simulink model "fft_overlap_tomori"  (R2023b)
settings: Solver=VariableStepAuto  StartTime=0.0  StopTime=inf  RelTol=1e-3
InitFcn:
  | fftparrallelout
  | load('dataram.mat')
  | s= fi(exp(-1j*2*pi.*(0:63)/64),1,16,15);
  | fixed_point = fixdt(1,27,20);
  | fixed_pointu = fixdt(0,29,20);
  | fixed = fixdt(1,22,15);
  | const = fixdt(1,18,17);
  | addConst = fixdt(1,18,16);
  | f =10.4e6;
  | f1=45e6;
  | alpha1 =5;
  | beta1 = 0.00001 ;
  | beta2 = 0.99999 ;
  | beta3 = 23;
undefined symbols (not defined in the file or in its folder): j
libraries: dspxfrm3 x11, commrflib2 x4
(part 8 of 10)

== system fft_overlap_tomori/FFT64_outMuxed/64pointFFTchan/FFT64/FFT32_1/complexmult4 ==
  x1 : Inport
  In3 : Inport  Port=2
  Add1 : Sum  OutDataTypeStr=addConst  RndMeth=Round
  Add2 : Sum  Inputs=+-  OutDataTypeStr=fixed  AccumDataTypeStr=fixed  RndMeth=Round
  Add20 : Sum  OutDataTypeStr=fixed  RndMeth=Round
  Add3 : Sum  Inputs=+-  OutDataTypeStr=fixed  AccumDataTypeStr=fixed  RndMeth=Round
  Add4 : Sum  Inputs=+-  OutDataTypeStr=fixed  AccumDataTypeStr=fixed  RndMeth=Round
  Complex to Real-Imag : ComplexToRealImag
  Complex to Real-Imag1 : ComplexToRealImag
  Constant : Constant  Commented=on  Value=1+j  OutDataTypeStr=fixdt(1,22, 15)  SampleTime=2e-8
  Constant1 : Constant  Commented=on  Value=1-j  OutDataTypeStr=fixdt(1,22, 15)  SampleTime=2e-8
  Data Type Conversion : DataTypeConversion  OutDataTypeStr=fixed  RndMeth=Round  SaturateOnIntegerOverflow=off
  Data Type Conversion1 : DataTypeConversion  OutDataTypeStr=fixed  RndMeth=Round  SaturateOnIntegerOverflow=off
  Data Type Conversion2 : DataTypeConversion  OutDataTypeStr=fixed  RndMeth=Round  SaturateOnIntegerOverflow=off
  Delay : Delay
  Delay1 : Delay
  Delay{3..14} (12 alike) : Delay  DelayLength=1
  Delay2 : Delay
  Display : Display  Commented=on
  Product : Product
  Product1 : Product
  Product2 : Product
  Real-Imag to Complex : RealImagToComplex
  Out1 : Outport
  wires:
  Real-Imag to Complex/1 -> Out1/1
  In3/1 -> Complex to Real-Imag1/1
  x1/1 -> Complex to Real-Imag/1
  Product/1 -> Delay/1
  Product1/1 -> Delay1/1
  Product2/1 -> Delay2/1
  Delay/1 -> Data Type Conversion/1
  Delay1/1 -> Data Type Conversion1/1
  Delay2/1 -> Data Type Conversion2/1
  Add4/1 -> Delay9/1
  Add3/1 -> Delay10/1
  Add20/1 -> Delay3/1
  Add1/1 -> Delay4/1
  Complex to Real-Imag/1 -> Delay5/1, Add20/1
  Complex to Real-Imag1/1 -> Delay6/1, Add1/1
  Complex to Real-Imag/2 -> Delay7/1, Add20/2
  Complex to Real-Imag1/2 -> Delay8/1, Add1/2
  Delay3/1 -> Product/1
  Delay4/1 -> Product/2
  Delay5/1 -> Product1/1
  Delay6/1 -> Product1/2
  Delay7/1 -> Product2/1
  Delay8/1 -> Product2/2
  Delay9/1 -> Real-Imag to Complex/1
  Delay10/1 -> Add2/1
  Delay11/1 -> Add2/2
  Add2/1 -> Real-Imag to Complex/2
  Delay12/1 -> Add3/1
  Data Type Conversion/1 -> Delay12/1
  Data Type Conversion1/1 -> Delay13/1
  Delay13/1 -> Add4/1, Add3/2
  Data Type Conversion2/1 -> Delay14/1
  Delay14/1 -> Delay11/1, Add4/2

== system fft_overlap_tomori/FFT64_outMuxed/64pointFFTchan/FFT64/FFT32_1/complexmult5 ==
  x1 : Inport
  In3 : Inport  Port=2
  Add1 : Sum  OutDataTypeStr=addConst  RndMeth=Round
  Add2 : Sum  Inputs=+-  OutDataTypeStr=fixed  AccumDataTypeStr=fixed  RndMeth=Round
  Add20 : Sum  OutDataTypeStr=fixed  RndMeth=Round
  Add3 : Sum  Inputs=+-  OutDataTypeStr=fixed  AccumDataTypeStr=fixed  RndMeth=Round
  Add4 : Sum  Inputs=+-  OutDataTypeStr=fixed  AccumDataTypeStr=fixed  RndMeth=Round
  Complex to Real-Imag : ComplexToRealImag
  Complex to Real-Imag1 : ComplexToRealImag
  Constant : Constant  Commented=on  Value=1+j  OutDataTypeStr=fixdt(1,22, 15)  SampleTime=2e-8
  Constant1 : Constant  Commented=on  Value=1-j  OutDataTypeStr=fixdt(1,22, 15)  SampleTime=2e-8
  Data Type Conversion : DataTypeConversion  OutDataTypeStr=fixed  RndMeth=Round  SaturateOnIntegerOverflow=off
  Data Type Conversion1 : DataTypeConversion  OutDataTypeStr=fixed  RndMeth=Round  SaturateOnIntegerOverflow=off
  Data Type Conversion2 : DataTypeConversion  OutDataTypeStr=fixed  RndMeth=Round  SaturateOnIntegerOverflow=off
  Delay : Delay
  Delay1 : Delay
  Delay{3..14} (12 alike) : Delay  DelayLength=1
  Delay2 : Delay
  Display : Display  Commented=on
  Product : Product
  Product1 : Product
  Product2 : Product
  Real-Imag to Complex : RealImagToComplex
  Out1 : Outport
  wires:
  Delay14/1 -> Add4/2, Delay11/1
  Data Type Conversion2/1 -> Delay14/1
  Delay13/1 -> Add3/2, Add4/1
  Data Type Conversion1/1 -> Delay13/1
  Data Type Conversion/1 -> Delay12/1
  Delay12/1 -> Add3/1
  Add2/1 -> Real-Imag to Complex/2
  Delay11/1 -> Add2/2
  Delay10/1 -> Add2/1
  Delay9/1 -> Real-Imag to Complex/1
  Delay8/1 -> Product2/2
  Delay7/1 -> Product2/1
  Delay6/1 -> Product1/2
  Delay5/1 -> Product1/1
  Delay4/1 -> Product/2
  Delay3/1 -> Product/1
  Complex to Real-Imag1/2 -> Add1/2, Delay8/1
  Complex to Real-Imag/2 -> Add20/2, Delay7/1
  Complex to Real-Imag1/1 -> Add1/1, Delay6/1
  Complex to Real-Imag/1 -> Add20/1, Delay5/1
  Add1/1 -> Delay4/1
  Add20/1 -> Delay3/1
  Add3/1 -> Delay10/1
  Add4/1 -> Delay9/1
  Delay2/1 -> Data Type Conversion2/1
  Delay1/1 -> Data Type Conversion1/1
  Delay/1 -> Data Type Conversion/1
  Product2/1 -> Delay2/1
  Product1/1 -> Delay1/1
  Product/1 -> Delay/1
  x1/1 -> Complex to Real-Imag/1
  In3/1 -> Complex to Real-Imag1/1
  Real-Imag to Complex/1 -> Out1/1

== system fft_overlap_tomori/FFT64_outMuxed/64pointFFTchan/FFT64/FFT32_1/complexmult6 ==
  x1 : Inport
  In3 : Inport  Port=2
  Add1 : Sum  OutDataTypeStr=addConst  RndMeth=Round
  Add2 : Sum  Inputs=+-  OutDataTypeStr=fixed  AccumDataTypeStr=fixed  RndMeth=Round
  Add20 : Sum  OutDataTypeStr=fixed  RndMeth=Round
  Add3 : Sum  Inputs=+-  OutDataTypeStr=fixed  AccumDataTypeStr=fixed  RndMeth=Round
  Add4 : Sum  Inputs=+-  OutDataTypeStr=fixed  AccumDataTypeStr=fixed  RndMeth=Round
  Complex to Real-Imag : ComplexToRealImag
  Complex to Real-Imag1 : ComplexToRealImag
  Constant : Constant  Commented=on  Value=1+j  OutDataTypeStr=fixdt(1,22, 15)  SampleTime=2e-8
  Constant1 : Constant  Commented=on  Value=1-j  OutDataTypeStr=fixdt(1,22, 15)  SampleTime=2e-8
  Data Type Conversion : DataTypeConversion  OutDataTypeStr=fixed  RndMeth=Round  SaturateOnIntegerOverflow=off
  Data Type Conversion1 : DataTypeConversion  OutDataTypeStr=fixed  RndMeth=Round  SaturateOnIntegerOverflow=off
  Data Type Conversion2 : DataTypeConversion  OutDataTypeStr=fixed  RndMeth=Round  SaturateOnIntegerOverflow=off
  Delay : Delay
  Delay1 : Delay
  Delay{3..14} (12 alike) : Delay  DelayLength=1
  Delay2 : Delay
  Display : Display  Commented=on
  Product : Product
  Product1 : Product
  Product2 : Product
  Real-Imag to Complex : RealImagToComplex
  Out1 : Outport
  wires:
  Real-Imag to Complex/1 -> Out1/1
  In3/1 -> Complex to Real-Imag1/1
  x1/1 -> Complex to Real-Imag/1
  Product/1 -> Delay/1
  Product1/1 -> Delay1/1
  Product2/1 -> Delay2/1
  Delay/1 -> Data Type Conversion/1
  Delay1/1 -> Data Type Conversion1/1
  Delay2/1 -> Data Type Conversion2/1
  Add4/1 -> Delay9/1
  Add3/1 -> Delay10/1
  Add20/1 -> Delay3/1
  Add1/1 -> Delay4/1
  Complex to Real-Imag/1 -> Delay5/1, Add20/1
  Complex to Real-Imag1/1 -> Delay6/1, Add1/1
  Complex to Real-Imag/2 -> Delay7/1, Add20/2
  Complex to Real-Imag1/2 -> Delay8/1, Add1/2
  Delay3/1 -> Product/1
  Delay4/1 -> Product/2
  Delay5/1 -> Product1/1
  Delay6/1 -> Product1/2
  Delay7/1 -> Product2/1
  Delay8/1 -> Product2/2
  Delay9/1 -> Real-Imag to Complex/1
  Delay10/1 -> Add2/1
  Delay11/1 -> Add2/2
  Add2/1 -> Real-Imag to Complex/2
  Delay12/1 -> Add3/1
  Data Type Conversion/1 -> Delay12/1
  Data Type Conversion1/1 -> Delay13/1
  Delay13/1 -> Add4/1, Add3/2
  Data Type Conversion2/1 -> Delay14/1
  Delay14/1 -> Delay11/1, Add4/2

== system fft_overlap_tomori/FFT64_outMuxed/64pointFFTchan/FFT64/FFT32_1/complexmult7 ==
  x1 : Inport
  In3 : Inport  Port=2
  Add1 : Sum  OutDataTypeStr=addConst  RndMeth=Round
  Add2 : Sum  Inputs=+-  OutDataTypeStr=fixed  AccumDataTypeStr=fixed  RndMeth=Round
  Add20 : Sum  OutDataTypeStr=fixed  RndMeth=Round
  Add3 : Sum  Inputs=+-  OutDataTypeStr=fixed  AccumDataTypeStr=fixed  RndMeth=Round
  Add4 : Sum  Inputs=+-  OutDataTypeStr=fixed  AccumDataTypeStr=fixed  RndMeth=Round
  Complex to Real-Imag : ComplexToRealImag
  Complex to Real-Imag1 : ComplexToRealImag
  Constant : Constant  Commented=on  Value=1+j  OutDataTypeStr=fixdt(1,22, 15)  SampleTime=2e-8
  Constant1 : Constant  Commented=on  Value=1-j  OutDataTypeStr=fixdt(1,22, 15)  SampleTime=2e-8
  Data Type Conversion : DataTypeConversion  OutDataTypeStr=fixed  RndMeth=Round  SaturateOnIntegerOverflow=off
  Data Type Conversion1 : DataTypeConversion  OutDataTypeStr=fixed  RndMeth=Round  SaturateOnIntegerOverflow=off
  Data Type Conversion2 : DataTypeConversion  OutDataTypeStr=fixed  RndMeth=Round  SaturateOnIntegerOverflow=off
  Delay : Delay
  Delay1 : Delay
  Delay{3..14} (12 alike) : Delay  DelayLength=1
  Delay2 : Delay
  Display : Display  Commented=on
  Product : Product
  Product1 : Product
  Product2 : Product
  Real-Imag to Complex : RealImagToComplex
  Out1 : Outport
  wires:
  Delay14/1 -> Add4/2, Delay11/1
  Data Type Conversion2/1 -> Delay14/1
  Delay13/1 -> Add3/2, Add4/1
  Data Type Conversion1/1 -> Delay13/1
  Data Type Conversion/1 -> Delay12/1
  Delay12/1 -> Add3/1
  Add2/1 -> Real-Imag to Complex/2
  Delay11/1 -> Add2/2
  Delay10/1 -> Add2/1
  Delay9/1 -> Real-Imag to Complex/1
  Delay8/1 -> Product2/2
  Delay7/1 -> Product2/1
  Delay6/1 -> Product1/2
  Delay5/1 -> Product1/1
  Delay4/1 -> Product/2
  Delay3/1 -> Product/1
  Complex to Real-Imag1/2 -> Add1/2, Delay8/1
  Complex to Real-Imag/2 -> Add20/2, Delay7/1
  Complex to Real-Imag1/1 -> Add1/1, Delay6/1
  Complex to Real-Imag/1 -> Add20/1, Delay5/1
  Add1/1 -> Delay4/1
  Add20/1 -> Delay3/1
  Add3/1 -> Delay10/1
  Add4/1 -> Delay9/1
  Delay2/1 -> Data Type Conversion2/1
  Delay1/1 -> Data Type Conversion1/1
  Delay/1 -> Data Type Conversion/1
  Product2/1 -> Delay2/1
  Product1/1 -> Delay1/1
  Product/1 -> Delay/1
  x1/1 -> Complex to Real-Imag/1
  In3/1 -> Complex to Real-Imag1/1
  Real-Imag to Complex/1 -> Out1/1

== system fft_overlap_tomori/FFT64_outMuxed/64pointFFTchan/FFT64/FFT32_1/complexmult8 ==
  x1 : Inport
  In3 : Inport  Port=2
  Add1 : Sum  OutDataTypeStr=addConst  RndMeth=Round
  Add2 : Sum  Inputs=+-  OutDataTypeStr=fixed  AccumDataTypeStr=fixed  RndMeth=Round
  Add20 : Sum  OutDataTypeStr=fixed  RndMeth=Round
  Add3 : Sum  Inputs=+-  OutDataTypeStr=fixed  AccumDataTypeStr=fixed  RndMeth=Round
  Add4 : Sum  Inputs=+-  OutDataTypeStr=fixed  AccumDataTypeStr=fixed  RndMeth=Round
  Complex to Real-Imag : ComplexToRealImag
  Complex to Real-Imag1 : ComplexToRealImag
  Constant : Constant  Commented=on  Value=1+j  OutDataTypeStr=fixdt(1,22, 15)  SampleTime=2e-8
  Constant1 : Constant  Commented=on  Value=1-j  OutDataTypeStr=fixdt(1,22, 15)  SampleTime=2e-8
  Data Type Conversion : DataTypeConversion  OutDataTypeStr=fixed  RndMeth=Round  SaturateOnIntegerOverflow=off
  Data Type Conversion1 : DataTypeConversion  OutDataTypeStr=fixed  RndMeth=Round  SaturateOnIntegerOverflow=off
  Data Type Conversion2 : DataTypeConversion  OutDataTypeStr=fixed  RndMeth=Round  SaturateOnIntegerOverflow=off
  Delay : Delay
  Delay1 : Delay
  Delay{3..14} (12 alike) : Delay  DelayLength=1
  Delay2 : Delay
  Display : Display  Commented=on
  Product : Product
  Product1 : Product
  Product2 : Product
  Real-Imag to Complex : RealImagToComplex
  Out1 : Outport
  wires:
  Real-Imag to Complex/1 -> Out1/1
  In3/1 -> Complex to Real-Imag1/1
  x1/1 -> Complex to Real-Imag/1
  Product/1 -> Delay/1
  Product1/1 -> Delay1/1
  Product2/1 -> Delay2/1
  Delay/1 -> Data Type Conversion/1
  Delay1/1 -> Data Type Conversion1/1
  Delay2/1 -> Data Type Conversion2/1
  Add4/1 -> Delay9/1
  Add3/1 -> Delay10/1
  Add20/1 -> Delay3/1
  Add1/1 -> Delay4/1
  Complex to Real-Imag/1 -> Delay5/1, Add20/1
  Complex to Real-Imag1/1 -> Delay6/1, Add1/1
  Complex to Real-Imag/2 -> Delay7/1, Add20/2
  Complex to Real-Imag1/2 -> Delay8/1, Add1/2
  Delay3/1 -> Product/1
  Delay4/1 -> Product/2
  Delay5/1 -> Product1/1
  Delay6/1 -> Product1/2
  Delay7/1 -> Product2/1
  Delay8/1 -> Product2/2
  Delay9/1 -> Real-Imag to Complex/1
  Delay10/1 -> Add2/1
  Delay11/1 -> Add2/2
  Add2/1 -> Real-Imag to Complex/2
  Delay12/1 -> Add3/1
  Data Type Conversion/1 -> Delay12/1
  Data Type Conversion1/1 -> Delay13/1
  Delay13/1 -> Add4/1, Add3/2
  Data Type Conversion2/1 -> Delay14/1
  Delay14/1 -> Delay11/1, Add4/2

== system fft_overlap_tomori/FFT64_outMuxed/64pointFFTchan/FFT64/FFT32_1/complexmult9 ==
  x1 : Inport
  In3 : Inport  Port=2
  Add1 : Sum  OutDataTypeStr=addConst  RndMeth=Round
  Add2 : Sum  Inputs=+-  OutDataTypeStr=fixed  AccumDataTypeStr=fixed  RndMeth=Round
  Add20 : Sum  OutDataTypeStr=fixed  RndMeth=Round
  Add3 : Sum  Inputs=+-  OutDataTypeStr=fixed  AccumDataTypeStr=fixed  RndMeth=Round
  Add4 : Sum  Inputs=+-  OutDataTypeStr=fixed  AccumDataTypeStr=fixed  RndMeth=Round
  Complex to Real-Imag : ComplexToRealImag
  Complex to Real-Imag1 : ComplexToRealImag
  Constant : Constant  Commented=on  Value=1+j  OutDataTypeStr=fixdt(1,22, 15)  SampleTime=2e-8
  Constant1 : Constant  Commented=on  Value=1-j  OutDataTypeStr=fixdt(1,22, 15)  SampleTime=2e-8
  Data Type Conversion : DataTypeConversion  OutDataTypeStr=fixed  RndMeth=Round  SaturateOnIntegerOverflow=off
  Data Type Conversion1 : DataTypeConversion  OutDataTypeStr=fixed  RndMeth=Round  SaturateOnIntegerOverflow=off
  Data Type Conversion2 : DataTypeConversion  OutDataTypeStr=fixed  RndMeth=Round  SaturateOnIntegerOverflow=off
  Delay : Delay
  Delay1 : Delay
  Delay{3..14} (12 alike) : Delay  DelayLength=1
  Delay2 : Delay
  Display : Display  Commented=on
  Product : Product
  Product1 : Product
  Product2 : Product
  Real-Imag to Complex : RealImagToComplex
  Out1 : Outport
  wires:
  Delay14/1 -> Add4/2, Delay11/1
  Data Type Conversion2/1 -> Delay14/1
  Delay13/1 -> Add3/2, Add4/1
  Data Type Conversion1/1 -> Delay13/1
  Data Type Conversion/1 -> Delay12/1
  Delay12/1 -> Add3/1
  Add2/1 -> Real-Imag to Complex/2
  Delay11/1 -> Add2/2
  Delay10/1 -> Add2/1
  Delay9/1 -> Real-Imag to Complex/1
  Delay8/1 -> Product2/2
  Delay7/1 -> Product2/1
  Delay6/1 -> Product1/2
  Delay5/1 -> Product1/1
  Delay4/1 -> Product/2
  Delay3/1 -> Product/1
  Complex to Real-Imag1/2 -> Add1/2, Delay8/1
  Complex to Real-Imag/2 -> Add20/2, Delay7/1
  Complex to Real-Imag1/1 -> Add1/1, Delay6/1
  Complex to Real-Imag/1 -> Add20/1, Delay5/1
  Add1/1 -> Delay4/1
  Add20/1 -> Delay3/1
  Add3/1 -> Delay10/1
  Add4/1 -> Delay9/1
  Delay2/1 -> Data Type Conversion2/1
  Delay1/1 -> Data Type Conversion1/1
  Delay/1 -> Data Type Conversion/1
  Product2/1 -> Delay2/1
  Product1/1 -> Delay1/1
  Product/1 -> Delay/1
  x1/1 -> Complex to Real-Imag/1
  In3/1 -> Complex to Real-Imag1/1
  Real-Imag to Complex/1 -> Out1/1

== system fft_overlap_tomori/FFT64_outMuxed/64pointFFTchan/FFT64/FFT32_1/multByExp(-j*Pi//4) ==
  x4 : Inport
  Add : Sum  OutDataTypeStr=fixed  RndMeth=Round
  Add1 : Sum  Inputs=+-  OutDataTypeStr=fixed  RndMeth=Round
  Complex to Real-Imag : ComplexToRealImag
  Data Type Conversion : DataTypeConversion  OutDataTypeStr=fixed  RndMeth=Round  SaturateOnIntegerOverflow=off
  Delay1 : Delay  DelayLength=1
  Delay24 : Delay  DelayLength=1
  Gain : Gain  Gain=sqrt(2)/2  ParamDataTypeStr=const
  Real-Imag to Complex : RealImagToComplex
  Out1 : Outport
  wires:
  x4/1 -> Gain/1
  Real-Imag to Complex/1 -> Out1/1
  Delay24/1 -> Complex to Real-Imag/1
  Add1/1 -> Real-Imag to Complex/2
  Add/1 -> Real-Imag to Complex/1
  Complex to Real-Imag/2 -> Add/2, Add1/1
  Complex to Real-Imag/1 -> Add/1, Add1/2
  Gain/1 -> Delay1/1
  Delay1/1 -> Data Type Conversion/1
  Data Type Conversion/1 -> Delay24/1

== system fft_overlap_tomori/FFT64_outMuxed/64pointFFTchan/FFT64/FFT32_1/multByExp(-j*Pi//4)1 ==
  x4 : Inport
  Add : Sum  OutDataTypeStr=fixed  RndMeth=Round
  Add1 : Sum  Inputs=+-  OutDataTypeStr=fixed  RndMeth=Round
  Complex to Real-Imag : ComplexToRealImag
  Data Type Conversion : DataTypeConversion  OutDataTypeStr=fixed  RndMeth=Round  SaturateOnIntegerOverflow=off
  Delay1 : Delay  DelayLength=1
  Delay24 : Delay  DelayLength=1
  Gain : Gain  Gain=sqrt(2)/2  ParamDataTypeStr=const
  Real-Imag to Complex : RealImagToComplex
  Out1 : Outport
  wires:
  x4/1 -> Gain/1
  Real-Imag to Complex/1 -> Out1/1
  Delay24/1 -> Complex to Real-Imag/1
  Add1/1 -> Real-Imag to Complex/2
  Add/1 -> Real-Imag to Complex/1
  Complex to Real-Imag/2 -> Add/2, Add1/1
  Complex to Real-Imag/1 -> Add/1, Add1/2
  Gain/1 -> Delay1/1
  Delay1/1 -> Data Type Conversion/1
  Data Type Conversion/1 -> Delay24/1

== system fft_overlap_tomori/FFT64_outMuxed/64pointFFTchan/FFT64/FFT32_1/multByMinusJ ==
  x4 : Inport
  Complex to Real-Imag : ComplexToRealImag
  Real-Imag to Complex : RealImagToComplex
  Unary Minus1 : UnaryMinus
  Out1 : Outport
  wires:
  Complex to Real-Imag/1 -> Unary Minus1/1
  Complex to Real-Imag/2 -> Real-Imag to Complex/1
  x4/1 -> Complex to Real-Imag/1
  Real-Imag to Complex/1 -> Out1/1
  Unary Minus1/1 -> Real-Imag to Complex/2

== system fft_overlap_tomori/FFT64_outMuxed/64pointFFTchan/FFT64/FFT32_1/multByMinusJ3 ==
  In1 : Inport
  Complex to Real-Imag : ComplexToRealImag
  Real-Imag to Complex : RealImagToComplex
  Unary Minus1 : UnaryMinus
  Out1 : Outport
  wires:
  Complex to Real-Imag/1 -> Unary Minus1/1
  Complex to Real-Imag/2 -> Real-Imag to Complex/1
  In1/1 -> Complex to Real-Imag/1
  Real-Imag to Complex/1 -> Out1/1
  Unary Minus1/1 -> Real-Imag to Complex/2

== system fft_overlap_tomori/16//32 and test junk/16pointfftchan1/fft_res/fft_1/proddd/s3 ==
  In1 : Inport
  Add16 : Sum  OutDataTypeStr=fixed_point  AccumDataTypeStr=fixed_point
  Add21 : Sum  Inputs=+-  OutDataTypeStr=fixed_point  AccumDataTypeStr=fixed_point
  Complex to Real-Imag : ComplexToRealImag
  Real-Imag to Complex : RealImagToComplex
  Out1 : Outport  VectorParamsAs1DForOutWhenUnconnected=off
  wires:
  Real-Imag to Complex/1 -> Out1/1
  In1/1 -> Complex to Real-Imag/1
  Complex to Real-Imag/1 -> Add21/2, Add16/1
  Complex to Real-Imag/2 -> Add21/1, Add16/2
  Add16/1 -> Real-Imag to Complex/1
  Add21/1 -> Real-Imag to Complex/2

== system fft_overlap_tomori/16//32 and test junk/16pointfftchan1/fft_res/fft_1/ptrrt/s4 ==
  In1 : Inport
  Add16 : Sum  OutDataTypeStr=fixed_point  AccumDataTypeStr=fixed_point
  Add21 : Sum  Inputs=+-  OutDataTypeStr=fixed_point  AccumDataTypeStr=fixed_point
  Complex to Real-Imag : ComplexToRealImag
  Real-Imag to Complex : RealImagToComplex
  Out1 : Outport  VectorParamsAs1DForOutWhenUnconnected=off
  wires:
  In1/1 -> Complex to Real-Imag/1
  Real-Imag to Complex/1 -> Out1/1
  Complex to Real-Imag/1 -> Add16/1, Add21/1
  Complex to Real-Imag/2 -> Add16/2, Add21/2
  Add21/1 -> Real-Imag to Complex/1
  Add16/1 -> Real-Imag to Complex/2

== system fft_overlap_tomori/16//32 and test junk/16pointfftchan1/fft_res/fft_8/proddd/s3 ==
  In1 : Inport
  Add16 : Sum  OutDataTypeStr=fixed_point  AccumDataTypeStr=fixed_point
  Add21 : Sum  Inputs=+-  OutDataTypeStr=fixed_point  AccumDataTypeStr=fixed_point
  Complex to Real-Imag : ComplexToRealImag
  Real-Imag to Complex : RealImagToComplex
  Out1 : Outport  VectorParamsAs1DForOutWhenUnconnected=off
  wires:
  Add21/1 -> Real-Imag to Complex/2
  Add16/1 -> Real-Imag to Complex/1
  Complex to Real-Imag/2 -> Add16/2, Add21/1
  Complex to Real-Imag/1 -> Add16/1, Add21/2
  In1/1 -> Complex to Real-Imag/1
  Real-Imag to Complex/1 -> Out1/1

== system fft_overlap_tomori/16//32 and test junk/16pointfftchan1/fft_res/fft_8/ptrrt/s4 ==
  In1 : Inport
  Add16 : Sum  OutDataTypeStr=fixed_point  AccumDataTypeStr=fixed_point
  Add21 : Sum  Inputs=+-  OutDataTypeStr=fixed_point  AccumDataTypeStr=fixed_point
  Complex to Real-Imag : ComplexToRealImag
  Real-Imag to Complex : RealImagToComplex
  Out1 : Outport  VectorParamsAs1DForOutWhenUnconnected=off
  wires:
  Add16/1 -> Real-Imag to Complex/2
  Add21/1 -> Real-Imag to Complex/1
  Complex to Real-Imag/2 -> Add21/2, Add16/2
  Complex to Real-Imag/1 -> Add21/1, Add16/1
  Real-Imag to Complex/1 -> Out1/1
  In1/1 -> Complex to Real-Imag/1

== system fft_overlap_tomori/16//32 and test junk/32/FFT32/FFT16/FFT8/multByExp(-j*Pi//4) ==
  In1 : Inport
  Add : Sum  OutDataTypeStr=fixed  RndMeth=Round
  Add1 : Sum  Inputs=+-  OutDataTypeStr=fixed  RndMeth=Round
  Complex to Real-Imag : ComplexToRealImag
  Delay24 : Delay
  Gain : Gain  Gain=sqrt(2)/2  ParamDataTypeStr=fixed  OutDataTypeStr=fixed  RndMeth=Round
  Real-Imag to Complex : RealImagToComplex
  Out1 : Outport
  wires:
  Real-Imag to Complex/1 -> Out1/1
  Gain/1 -> Delay24/1
  Complex to Real-Imag/1 -> Add1/2, Add/1
  Complex to Real-Imag/2 -> Add1/1, Add/2
  Add/1 -> Real-Imag to Complex/1
  Add1/1 -> Real-Imag to Complex/2
  Delay24/1 -> Complex to Real-Imag/1
  In1/1 -> Gain/1

== system fft_overlap_tomori/16//32 and test junk/32/FFT32/FFT16/FFT8/multByExp(-j*Pi//4)1 ==
  In1 : Inport
  Add : Sum  OutDataTypeStr=fixed  RndMeth=Round
  Add1 : Sum  Inputs=+-  OutDataTypeStr=fixed  RndMeth=Round
  Complex to Real-Imag : ComplexToRealImag
  Delay24 : Delay
  Gain : Gain  Gain=sqrt(2)/2  ParamDataTypeStr=fixed  OutDataTypeStr=fixed  RndMeth=Round
  Real-Imag to Complex : RealImagToComplex
  Out1 : Outport
  wires:
  Real-Imag to Complex/1 -> Out1/1
  Gain/1 -> Delay24/1
  Complex to Real-Imag/1 -> Add1/2, Add/1
  Complex to Real-Imag/2 -> Add1/1, Add/2
  Add/1 -> Real-Imag to Complex/1
  Add1/1 -> Real-Imag to Complex/2
  Delay24/1 -> Complex to Real-Imag/1
  In1/1 -> Gain/1

== system fft_overlap_tomori/16//32 and test junk/32/FFT32/FFT16/FFT8/multByMinusJ ==
  In1 : Inport
  Complex to Real-Imag : ComplexToRealImag
  Real-Imag to Complex : RealImagToComplex
  Unary Minus1 : UnaryMinus
  Out1 : Outport
  wires:
  Complex to Real-Imag/1 -> Unary Minus1/1
  Complex to Real-Imag/2 -> Real-Imag to Complex/1
  In1/1 -> Complex to Real-Imag/1
  Real-Imag to Complex/1 -> Out1/1
  Unary Minus1/1 -> Real-Imag to Complex/2

== system fft_overlap_tomori/16//32 and test junk/32/FFT32/FFT16/FFT8/multByMinusJ1 ==
  In1 : Inport
  Complex to Real-Imag : ComplexToRealImag
  Real-Imag to Complex : RealImagToComplex
  Unary Minus1 : UnaryMinus
  Out1 : Outport
  wires:
  Unary Minus1/1 -> Real-Imag to Complex/2
  Real-Imag to Complex/1 -> Out1/1
  In1/1 -> Complex to Real-Imag/1
  Complex to Real-Imag/2 -> Real-Imag to Complex/1
  Complex to Real-Imag/1 -> Unary Minus1/1

== system fft_overlap_tomori/16//32 and test junk/32/FFT32/FFT16/FFT8/multByMinusJ2 ==
  In1 : Inport
  Complex to Real-Imag : ComplexToRealImag
  Real-Imag to Complex : RealImagToComplex
  Unary Minus1 : UnaryMinus
  Out1 : Outport
  wires:
  Unary Minus1/1 -> Real-Imag to Complex/2
  Real-Imag to Complex/1 -> Out1/1
  In1/1 -> Complex to Real-Imag/1
  Complex to Real-Imag/2 -> Real-Imag to Complex/1
  Complex to Real-Imag/1 -> Unary Minus1/1

== system fft_overlap_tomori/16//32 and test junk/32/FFT32/FFT16/FFT8/multByMinusJ3 ==
  In1 : Inport
  Complex to Real-Imag : ComplexToRealImag
  Real-Imag to Complex : RealImagToComplex
  Unary Minus1 : UnaryMinus
  Out1 : Outport
  wires:
  Complex to Real-Imag/1 -> Unary Minus1/1
  Complex to Real-Imag/2 -> Real-Imag to Complex/1
  In1/1 -> Complex to Real-Imag/1
  Real-Imag to Complex/1 -> Out1/1
  Unary Minus1/1 -> Real-Imag to Complex/2

== system fft_overlap_tomori/16//32 and test junk/32/FFT32/FFT16/FFT8_1/multByExp(-j*Pi//4) ==
  In1 : Inport
  Add : Sum  OutDataTypeStr=fixed  RndMeth=Round
  Add1 : Sum  Inputs=+-  OutDataTypeStr=fixed  RndMeth=Round
  Complex to Real-Imag : ComplexToRealImag
  Delay24 : Delay
  Gain : Gain  Gain=sqrt(2)/2  ParamDataTypeStr=fixed  OutDataTypeStr=fixed  RndMeth=Round
  Real-Imag to Complex : RealImagToComplex
  Out1 : Outport
  wires:
  Real-Imag to Complex/1 -> Out1/1
  Gain/1 -> Delay24/1
  Complex to Real-Imag/1 -> Add1/2, Add/1
  Complex to Real-Imag/2 -> Add1/1, Add/2
  Add/1 -> Real-Imag to Complex/1
  Add1/1 -> Real-Imag to Complex/2
  Delay24/1 -> Complex to Real-Imag/1
  In1/1 -> Gain/1

== system fft_overlap_tomori/16//32 and test junk/32/FFT32/FFT16/FFT8_1/multByExp(-j*Pi//4)1 ==
  In1 : Inport
  Add : Sum  OutDataTypeStr=fixed  RndMeth=Round
  Add1 : Sum  Inputs=+-  OutDataTypeStr=fixed  RndMeth=Round
  Complex to Real-Imag : ComplexToRealImag
  Delay24 : Delay
  Gain : Gain  Gain=sqrt(2)/2  ParamDataTypeStr=fixed  OutDataTypeStr=fixed  RndMeth=Round
  Real-Imag to Complex : RealImagToComplex
  Out1 : Outport
  wires:
  Real-Imag to Complex/1 -> Out1/1
  Gain/1 -> Delay24/1
  Complex to Real-Imag/1 -> Add1/2, Add/1
  Complex to Real-Imag/2 -> Add1/1, Add/2
  Add/1 -> Real-Imag to Complex/1
  Add1/1 -> Real-Imag to Complex/2
  Delay24/1 -> Complex to Real-Imag/1
  In1/1 -> Gain/1

== system fft_overlap_tomori/16//32 and test junk/32/FFT32/FFT16/FFT8_1/multByMinusJ ==
  In1 : Inport
  Complex to Real-Imag : ComplexToRealImag
  Real-Imag to Complex : RealImagToComplex
  Unary Minus1 : UnaryMinus
  Out1 : Outport
  wires:
  Complex to Real-Imag/1 -> Unary Minus1/1
  Complex to Real-Imag/2 -> Real-Imag to Complex/1
  In1/1 -> Complex to Real-Imag/1
  Real-Imag to Complex/1 -> Out1/1
  Unary Minus1/1 -> Real-Imag to Complex/2

== system fft_overlap_tomori/16//32 and test junk/32/FFT32/FFT16/FFT8_1/multByMinusJ1 ==
  In1 : Inport
  Complex to Real-Imag : ComplexToRealImag
  Real-Imag to Complex : RealImagToComplex
  Unary Minus1 : UnaryMinus
  Out1 : Outport
  wires:
  Unary Minus1/1 -> Real-Imag to Complex/2
  Real-Imag to Complex/1 -> Out1/1
  In1/1 -> Complex to Real-Imag/1
  Complex to Real-Imag/2 -> Real-Imag to Complex/1
  Complex to Real-Imag/1 -> Unary Minus1/1

== system fft_overlap_tomori/16//32 and test junk/32/FFT32/FFT16/FFT8_1/multByMinusJ2 ==
  In1 : Inport
  Complex to Real-Imag : ComplexToRealImag
  Real-Imag to Complex : RealImagToComplex
  Unary Minus1 : UnaryMinus
  Out1 : Outport
  wires:
  Unary Minus1/1 -> Real-Imag to Complex/2
  Real-Imag to Complex/1 -> Out1/1
  In1/1 -> Complex to Real-Imag/1
  Complex to Real-Imag/2 -> Real-Imag to Complex/1
  Complex to Real-Imag/1 -> Unary Minus1/1

== system fft_overlap_tomori/16//32 and test junk/32/FFT32/FFT16/FFT8_1/multByMinusJ3 ==
  In1 : Inport
  Complex to Real-Imag : ComplexToRealImag
  Real-Imag to Complex : RealImagToComplex
  Unary Minus1 : UnaryMinus
  Out1 : Outport
  wires:
  Complex to Real-Imag/1 -> Unary Minus1/1
  Complex to Real-Imag/2 -> Real-Imag to Complex/1
  In1/1 -> Complex to Real-Imag/1
  Real-Imag to Complex/1 -> Out1/1
  Unary Minus1/1 -> Real-Imag to Complex/2

== system fft_overlap_tomori/16//32 and test junk/32/FFT32/FFT16_1/FFT8/multByExp(-j*Pi//4) ==
  In1 : Inport
  Add : Sum  OutDataTypeStr=fixed  RndMeth=Round
  Add1 : Sum  Inputs=+-  OutDataTypeStr=fixed  RndMeth=Round
  Complex to Real-Imag : ComplexToRealImag
  Delay24 : Delay
  Gain : Gain  Gain=sqrt(2)/2  ParamDataTypeStr=fixed  OutDataTypeStr=fixed  RndMeth=Round
  Real-Imag to Complex : RealImagToComplex
  Out1 : Outport
  wires:
  In1/1 -> Gain/1
  Delay24/1 -> Complex to Real-Imag/1
  Add1/1 -> Real-Imag to Complex/2
  Add/1 -> Real-Imag to Complex/1
  Complex to Real-Imag/2 -> Add/2, Add1/1
  Complex to Real-Imag/1 -> Add/1, Add1/2
  Gain/1 -> Delay24/1
  Real-Imag to Complex/1 -> Out1/1

== system fft_overlap_tomori/16//32 and test junk/32/FFT32/FFT16_1/FFT8/multByExp(-j*Pi//4)1 ==
  In1 : Inport
  Add : Sum  OutDataTypeStr=fixed  RndMeth=Round
  Add1 : Sum  Inputs=+-  OutDataTypeStr=fixed  RndMeth=Round
  Complex to Real-Imag : ComplexToRealImag
  Delay24 : Delay
  Gain : Gain  Gain=sqrt(2)/2  ParamDataTypeStr=fixed  OutDataTypeStr=fixed  RndMeth=Round
  Real-Imag to Complex : RealImagToComplex
  Out1 : Outport
  wires:
  In1/1 -> Gain/1
  Delay24/1 -> Complex to Real-Imag/1
  Add1/1 -> Real-Imag to Complex/2
  Add/1 -> Real-Imag to Complex/1
  Complex to Real-Imag/2 -> Add/2, Add1/1
  Complex to Real-Imag/1 -> Add/1, Add1/2
  Gain/1 -> Delay24/1
  Real-Imag to Complex/1 -> Out1/1

== system fft_overlap_tomori/16//32 and test junk/32/FFT32/FFT16_1/FFT8/multByMinusJ ==
  In1 : Inport
  Complex to Real-Imag : ComplexToRealImag
  Real-Imag to Complex : RealImagToComplex
  Unary Minus1 : UnaryMinus
  Out1 : Outport
  wires:
  Unary Minus1/1 -> Real-Imag to Complex/2
  Real-Imag to Complex/1 -> Out1/1
  In1/1 -> Complex to Real-Imag/1
  Complex to Real-Imag/2 -> Real-Imag to Complex/1
  Complex to Real-Imag/1 -> Unary Minus1/1

== system fft_overlap_tomori/16//32 and test junk/32/FFT32/FFT16_1/FFT8/multByMinusJ1 ==
  In1 : Inport
  Complex to Real-Imag : ComplexToRealImag
  Real-Imag to Complex : RealImagToComplex
  Unary Minus1 : UnaryMinus
  Out1 : Outport
  wires:
  Complex to Real-Imag/1 -> Unary Minus1/1
  Complex to Real-Imag/2 -> Real-Imag to Complex/1
  In1/1 -> Complex to Real-Imag/1
  Real-Imag to Complex/1 -> Out1/1
  Unary Minus1/1 -> Real-Imag to Complex/2

== system fft_overlap_tomori/16//32 and test junk/32/FFT32/FFT16_1/FFT8/multByMinusJ2 ==
  In1 : Inport
  Complex to Real-Imag : ComplexToRealImag
  Real-Imag to Complex : RealImagToComplex
  Unary Minus1 : UnaryMinus
  Out1 : Outport
  wires:
  Complex to Real-Imag/1 -> Unary Minus1/1
  Complex to Real-Imag/2 -> Real-Imag to Complex/1
  In1/1 -> Complex to Real-Imag/1
  Real-Imag to Complex/1 -> Out1/1
  Unary Minus1/1 -> Real-Imag to Complex/2

== system fft_overlap_tomori/16//32 and test junk/32/FFT32/FFT16_1/FFT8/multByMinusJ3 ==
  In1 : Inport
  Complex to Real-Imag : ComplexToRealImag
  Real-Imag to Complex : RealImagToComplex
  Unary Minus1 : UnaryMinus
  Out1 : Outport
  wires:
  Unary Minus1/1 -> Real-Imag to Complex/2
  Real-Imag to Complex/1 -> Out1/1
  In1/1 -> Complex to Real-Imag/1
  Complex to Real-Imag/2 -> Real-Imag to Complex/1
  Complex to Real-Imag/1 -> Unary Minus1/1

== system fft_overlap_tomori/16//32 and test junk/32/FFT32/FFT16_1/FFT8_1/multByExp(-j*Pi//4) ==
  In1 : Inport
  Add : Sum  OutDataTypeStr=fixed  RndMeth=Round
  Add1 : Sum  Inputs=+-  OutDataTypeStr=fixed  RndMeth=Round
  Complex to Real-Imag : ComplexToRealImag
  Delay24 : Delay
  Gain : Gain  Gain=sqrt(2)/2  ParamDataTypeStr=fixed  OutDataTypeStr=fixed  RndMeth=Round
  Real-Imag to Complex : RealImagToComplex
  Out1 : Outport
  wires:
  In1/1 -> Gain/1
  Delay24/1 -> Complex to Real-Imag/1
  Add1/1 -> Real-Imag to Complex/2
  Add/1 -> Real-Imag to Complex/1
  Complex to Real-Imag/2 -> Add/2, Add1/1
  Complex to Real-Imag/1 -> Add/1, Add1/2
  Gain/1 -> Delay24/1
  Real-Imag to Complex/1 -> Out1/1

== system fft_overlap_tomori/16//32 and test junk/32/FFT32/FFT16_1/FFT8_1/multByExp(-j*Pi//4)1 ==
  In1 : Inport
  Add : Sum  OutDataTypeStr=fixed  RndMeth=Round
  Add1 : Sum  Inputs=+-  OutDataTypeStr=fixed  RndMeth=Round
  Complex to Real-Imag : ComplexToRealImag
  Delay24 : Delay
  Gain : Gain  Gain=sqrt(2)/2  ParamDataTypeStr=fixed  OutDataTypeStr=fixed  RndMeth=Round
  Real-Imag to Complex : RealImagToComplex
  Out1 : Outport
  wires:
  In1/1 -> Gain/1
  Delay24/1 -> Complex to Real-Imag/1
  Add1/1 -> Real-Imag to Complex/2
  Add/1 -> Real-Imag to Complex/1
  Complex to Real-Imag/2 -> Add/2, Add1/1
  Complex to Real-Imag/1 -> Add/1, Add1/2
  Gain/1 -> Delay24/1
  Real-Imag to Complex/1 -> Out1/1

== system fft_overlap_tomori/16//32 and test junk/32/FFT32/FFT16_1/FFT8_1/multByMinusJ ==
  In1 : Inport
  Complex to Real-Imag : ComplexToRealImag
  Real-Imag to Complex : RealImagToComplex
  Unary Minus1 : UnaryMinus
  Out1 : Outport
  wires:
  Unary Minus1/1 -> Real-Imag to Complex/2
  Real-Imag to Complex/1 -> Out1/1
  In1/1 -> Complex to Real-Imag/1
  Complex to Real-Imag/2 -> Real-Imag to Complex/1
  Complex to Real-Imag/1 -> Unary Minus1/1

== system fft_overlap_tomori/16//32 and test junk/32/FFT32/FFT16_1/FFT8_1/multByMinusJ1 ==
  In1 : Inport
  Complex to Real-Imag : ComplexToRealImag
  Real-Imag to Complex : RealImagToComplex
  Unary Minus1 : UnaryMinus
  Out1 : Outport
  wires:
  Complex to Real-Imag/1 -> Unary Minus1/1
  Complex to Real-Imag/2 -> Real-Imag to Complex/1
  In1/1 -> Complex to Real-Imag/1
  Real-Imag to Complex/1 -> Out1/1
  Unary Minus1/1 -> Real-Imag to Complex/2

== system fft_overlap_tomori/16//32 and test junk/32/FFT32/FFT16_1/FFT8_1/multByMinusJ2 ==
  In1 : Inport
  Complex to Real-Imag : ComplexToRealImag
  Real-Imag to Complex : RealImagToComplex
  Unary Minus1 : UnaryMinus
  Out1 : Outport
  wires:
  Complex to Real-Imag/1 -> Unary Minus1/1
  Complex to Real-Imag/2 -> Real-Imag to Complex/1
  In1/1 -> Complex to Real-Imag/1
  Real-Imag to Complex/1 -> Out1/1
  Unary Minus1/1 -> Real-Imag to Complex/2

== system fft_overlap_tomori/16//32 and test junk/32/FFT32/FFT16_1/FFT8_1/multByMinusJ3 ==
  In1 : Inport
  Complex to Real-Imag : ComplexToRealImag
  Real-Imag to Complex : RealImagToComplex
  Unary Minus1 : UnaryMinus
  Out1 : Outport
  wires:
  Unary Minus1/1 -> Real-Imag to Complex/2
  Real-Imag to Complex/1 -> Out1/1
  In1/1 -> Complex to Real-Imag/1
  Complex to Real-Imag/2 -> Real-Imag to Complex/1
  Complex to Real-Imag/1 -> Unary Minus1/1

== system fft_overlap_tomori/FFT64_outMuxed/64pointFFTchan/FFT64/FFT32/FFT16/FFT8 ==
  In1 : Inport
  In2 : Inport  Port=2
  In3 : Inport  Port=3
  In4 : Inport  Port=4
  In5 : Inport  Port=5
  In6 : Inport  Port=6
  In7 : Inport  Port=7
  In8 : Inport  Port=8
  Add{,2,4,6,8,10,12,14,16,18,20,22} (12 alike) : Sum  OutDataTypeStr=fixed  RndMeth=Round
  Add{1,3,5,7,9,11,13,15,17,19,21,23} (12 alike) : Sum  Inputs=+-  OutDataTypeStr=fixed  RndMeth=Round
  Delay{,1,4..9,16..17} (10 alike) : Delay  DelayLength=1
  Delay{2..3,10..15,18..23} (14 alike) : Delay  DelayLength=3
  Delay{24..31} (8 alike) : Delay
  multByExp(-j*Pi/4) : Subsystem
  multByExp(-j*Pi/4)1 : Subsystem
  multByMinusJ : Subsystem
  multByMinusJ1 : Subsystem
  multByMinusJ2 : Subsystem
  multByMinusJ3 : Subsystem
  x0 : Outport
  x1 : Outport  Port=2  VectorParamsAs1DForOutWhenUnconnected=off
  x2 : Outport  Port=3  VectorParamsAs1DForOutWhenUnconnected=off
  x3 : Outport  Port=4  VectorParamsAs1DForOutWhenUnconnected=off
  x4 : Outport  Port=5  VectorParamsAs1DForOutWhenUnconnected=off
  x5 : Outport  Port=6  VectorParamsAs1DForOutWhenUnconnected=off
  x6 : Outport  Port=7  VectorParamsAs1DForOutWhenUnconnected=off
  x7 : Outport  Port=8  VectorParamsAs1DForOutWhenUnconnected=off
  wires:
  Delay17/1 -> Add21/2, Add20/2
  Delay15/1 -> Add21/1, Add20/1
  Delay23/1 -> x7/1
  Delay22/1 -> x3/1
  Delay21/1 -> x5/1
  Delay20/1 -> x1/1
  multByExp(-j*Pi/4)1/1(Out1) -> multByMinusJ3/1(In1)
  multByExp(-j*Pi/4)/1(Out1) -> Delay16/1
  multByMinusJ3/1(Out1) -> Delay17/1
  Delay16/1 -> Add18/2, Add19/2
  Delay14/1 -> Add19/1, Add18/1
  Add21/1 -> Delay23/1
  Add20/1 -> Delay22/1
  Add19/1 -> Delay21/1
  Add18/1 -> Delay20/1
  Delay19/1 -> x6/1
  Delay18/1 -> x2/1
  Delay11/1 -> Add12/2, Add13/2
  multByMinusJ2/1(Out1) -> Delay11/1
  Add13/1 -> Delay19/1
  Add12/1 -> Delay18/1
  Delay3/1 -> Add13/1, Add12/1
  Add17/1 -> Delay24/1
  Add16/1 -> Delay25/1
  Delay9/1 -> Add16/2, Add17/2
  Delay5/1 -> Add16/1, Add17/1
  multByMinusJ1/1(Out1) -> Delay9/1
  multByMinusJ/1(Out1) -> Delay7/1
  Add15/1 -> Delay26/1
  Add14/1 -> Delay27/1
  Delay7/1 -> Add15/2, Add14/2
  Delay1/1 -> Add15/1, Add14/1
  Delay13/1 -> x4/1
  Delay12/1 -> x0/1
  Add23/1 -> Delay13/1
  Add22/1 -> Delay12/1
  Delay10/1 -> Add22/2, Add23/2
  Delay2/1 -> Add23/1, Add22/1
  Delay6/1 -> Add3/2, Add2/2
  Add11/1 -> Delay28/1
  Add10/1 -> Delay29/1
  Delay8/1 -> Add10/2, Add11/2
  Delay4/1 -> Add11/1, Add10/1
  Add9/1 -> multByMinusJ1/1(In1)
  Add8/1 -> Delay8/1
  Add7/1 -> multByMinusJ/1(In1)
  Add6/1 -> Delay6/1
  Add5/1 -> Delay5/1
  Add4/1 -> Delay4/1
  In8/1 -> Add9/2, Add8/2
  In4/1 -> Add8/1, Add9/1
  In6/1 -> Add5/2, Add4/2
  In2/1 -> Add4/1, Add5/1
  In7/1 -> Add7/2, Add6/2
  In3/1 -> Add6/1, Add7/1
  Add3/1 -> Delay30/1
  Add2/1 -> Delay31/1
  Delay/1 -> Add3/1, Add2/1
  Add1/1 -> Delay1/1
  Add/1 -> Delay/1
  In5/1 -> Add1/2, Add/2
  In1/1 -> Add/1, Add1/1
  Delay24/1 -> multByExp(-j*Pi/4)1/1(x4)
  Delay25/1 -> multByExp(-j*Pi/4)/1(x4)
  Delay26/1 -> Delay15/1
  Delay27/1 -> Delay14/1
  Delay28/1 -> multByMinusJ2/1(In1)
  Delay29/1 -> Delay10/1
  Delay30/1 -> Delay3/1
  Delay31/1 -> Delay2/1

== system fft_overlap_tomori/FFT64_outMuxed/64pointFFTchan/FFT64/FFT32/FFT16/FFT8_1 ==
  In1 : Inport
  In2 : Inport  Port=2
  In3 : Inport  Port=3
  In4 : Inport  Port=4
  In5 : Inport  Port=5
  In6 : Inport  Port=6
  In7 : Inport  Port=7
  In8 : Inport  Port=8
  Add{,2,4,6,8,10,12,14,16,18,20,22} (12 alike) : Sum  OutDataTypeStr=fixed  RndMeth=Round
  Add{1,3,5,7,9,11,13,15,17,19,21,23} (12 alike) : Sum  Inputs=+-  OutDataTypeStr=fixed  RndMeth=Round
  Delay{,1,4..9,16..17} (10 alike) : Delay  DelayLength=1
  Delay{2..3,10..15,18..23} (14 alike) : Delay  DelayLength=3
  Delay{24..31} (8 alike) : Delay
  multByExp(-j*Pi/4) : Subsystem
  multByExp(-j*Pi/4)1 : Subsystem
  multByMinusJ : Subsystem
  multByMinusJ1 : Subsystem
  multByMinusJ2 : Subsystem
  multByMinusJ3 : Subsystem
  x0 : Outport
  x1 : Outport  Port=2  VectorParamsAs1DForOutWhenUnconnected=off
  x2 : Outport  Port=3  VectorParamsAs1DForOutWhenUnconnected=off
  x3 : Outport  Port=4  VectorParamsAs1DForOutWhenUnconnected=off
  x4 : Outport  Port=5  VectorParamsAs1DForOutWhenUnconnected=off
  x5 : Outport  Port=6  VectorParamsAs1DForOutWhenUnconnected=off
  x6 : Outport  Port=7  VectorParamsAs1DForOutWhenUnconnected=off
  x7 : Outport  Port=8  VectorParamsAs1DForOutWhenUnconnected=off
  wires:
  Delay31/1 -> Delay2/1
  Delay30/1 -> Delay3/1
  Delay29/1 -> Delay10/1
  Delay28/1 -> multByMinusJ2/1(In1)
  Delay27/1 -> Delay14/1
  Delay26/1 -> Delay15/1
  Delay25/1 -> multByExp(-j*Pi/4)/1(x4)
  Delay24/1 -> multByExp(-j*Pi/4)1/1(x4)
  In1/1 -> Add1/1, Add/1
  In5/1 -> Add/2, Add1/2
  Add/1 -> Delay/1
  Add1/1 -> Delay1/1
  Delay/1 -> Add2/1, Add3/1
  Add2/1 -> Delay31/1
  Add3/1 -> Delay30/1
  In3/1 -> Add7/1, Add6/1
  In7/1 -> Add6/2, Add7/2
  In2/1 -> Add5/1, Add4/1
  In6/1 -> Add4/2, Add5/2
  In4/1 -> Add9/1, Add8/1
  In8/1 -> Add8/2, Add9/2
  Add4/1 -> Delay4/1
  Add5/1 -> Delay5/1
  Add6/1 -> Delay6/1
  Add7/1 -> multByMinusJ/1(In1)
  Add8/1 -> Delay8/1
  Add9/1 -> multByMinusJ1/1(In1)
  Delay4/1 -> Add10/1, Add11/1
  Delay8/1 -> Add11/2, Add10/2
  Add10/1 -> Delay29/1
  Add11/1 -> Delay28/1
  Delay6/1 -> Add2/2, Add3/2
  Delay2/1 -> Add22/1, Add23/1
  Delay10/1 -> Add23/2, Add22/2
  Add22/1 -> Delay12/1
  Add23/1 -> Delay13/1
  Delay12/1 -> x0/1
  Delay13/1 -> x4/1
  Delay1/1 -> Add14/1, Add15/1
  Delay7/1 -> Add14/2, Add15/2
  Add14/1 -> Delay27/1
  Add15/1 -> Delay26/1
  multByMinusJ/1(Out1) -> Delay7/1
  multByMinusJ1/1(Out1) -> Delay9/1
  Delay5/1 -> Add17/1, Add16/1
  Delay9/1 -> Add17/2, Add16/2
  Add16/1 -> Delay25/1
  Add17/1 -> Delay24/1
  Delay3/1 -> Add12/1, Add13/1
  Add12/1 -> Delay18/1
  Add13/1 -> Delay19/1
  multByMinusJ2/1(Out1) -> Delay11/1
  Delay11/1 -> Add13/2, Add12/2
  Delay18/1 -> x2/1
  Delay19/1 -> x6/1
  Add18/1 -> Delay20/1
  Add19/1 -> Delay21/1
  Add20/1 -> Delay22/1
  Add21/1 -> Delay23/1
  Delay14/1 -> Add18/1, Add19/1
  Delay16/1 -> Add19/2, Add18/2
  multByMinusJ3/1(Out1) -> Delay17/1
  multByExp(-j*Pi/4)/1(Out1) -> Delay16/1
  multByExp(-j*Pi/4)1/1(Out1) -> multByMinusJ3/1(In1)
  Delay20/1 -> x1/1
  Delay21/1 -> x5/1
  Delay22/1 -> x3/1
  Delay23/1 -> x7/1
  Delay15/1 -> Add20/1, Add21/1
  Delay17/1 -> Add20/2, Add21/2

== system fft_overlap_tomori/FFT64_outMuxed/64pointFFTchan/FFT64/FFT32/FFT16/complexmult ==
  x1 : Inport
  In3 : Inport  Port=2
  Add1 : Sum  OutDataTypeStr=addConst  RndMeth=Round
  Add2 : Sum  Inputs=+-  OutDataTypeStr=fixed  AccumDataTypeStr=fixed  RndMeth=Round
  Add20 : Sum  OutDataTypeStr=fixed  RndMeth=Round
  Add3 : Sum  Inputs=+-  OutDataTypeStr=fixed  AccumDataTypeStr=fixed  RndMeth=Round
  Add4 : Sum  Inputs=+-  OutDataTypeStr=fixed  AccumDataTypeStr=fixed  RndMeth=Round
  Complex to Real-Imag : ComplexToRealImag
  Complex to Real-Imag1 : ComplexToRealImag
  Constant : Constant  Commented=on  Value=1+j  OutDataTypeStr=fixdt(1,22, 15)  SampleTime=2e-8
  Constant1 : Constant  Commented=on  Value=1-j  OutDataTypeStr=fixdt(1,22, 15)  SampleTime=2e-8
  Data Type Conversion : DataTypeConversion  OutDataTypeStr=fixed  RndMeth=Round  SaturateOnIntegerOverflow=off
  Data Type Conversion1 : DataTypeConversion  OutDataTypeStr=fixed  RndMeth=Round  SaturateOnIntegerOverflow=off
  Data Type Conversion2 : DataTypeConversion  OutDataTypeStr=fixed  RndMeth=Round  SaturateOnIntegerOverflow=off
  Delay : Delay
  Delay1 : Delay
  Delay{3..14} (12 alike) : Delay  DelayLength=1
  Delay2 : Delay
  Display : Display  Commented=on
  Product : Product
  Product1 : Product
  Product2 : Product
  Real-Imag to Complex : RealImagToComplex
  Out1 : Outport
  wires:
  Real-Imag to Complex/1 -> Out1/1
  In3/1 -> Complex to Real-Imag1/1
  x1/1 -> Complex to Real-Imag/1
  Product/1 -> Delay/1
  Product1/1 -> Delay1/1
  Product2/1 -> Delay2/1
  Delay/1 -> Data Type Conversion/1
  Delay1/1 -> Data Type Conversion1/1
  Delay2/1 -> Data Type Conversion2/1
  Add4/1 -> Delay9/1
  Add3/1 -> Delay10/1
  Add20/1 -> Delay3/1
  Add1/1 -> Delay4/1
  Complex to Real-Imag/1 -> Delay5/1, Add20/1
  Complex to Real-Imag1/1 -> Delay6/1, Add1/1
  Complex to Real-Imag/2 -> Delay7/1, Add20/2
  Complex to Real-Imag1/2 -> Delay8/1, Add1/2
  Delay3/1 -> Product/1
  Delay4/1 -> Product/2
  Delay5/1 -> Product1/1
  Delay6/1 -> Product1/2
  Delay7/1 -> Product2/1
  Delay8/1 -> Product2/2
  Delay9/1 -> Real-Imag to Complex/1
  Delay10/1 -> Add2/1
  Delay11/1 -> Add2/2
  Add2/1 -> Real-Imag to Complex/2
  Delay12/1 -> Add3/1
  Data Type Conversion/1 -> Delay12/1
  Data Type Conversion1/1 -> Delay13/1
  Delay13/1 -> Add4/1, Add3/2
  Data Type Conversion2/1 -> Delay14/1
  Delay14/1 -> Delay11/1, Add4/2

== system fft_overlap_tomori/FFT64_outMuxed/64pointFFTchan/FFT64/FFT32/FFT16/complexmult1 ==
  x1 : Inport
  In3 : Inport  Port=2
  Add1 : Sum  OutDataTypeStr=addConst  RndMeth=Round
  Add2 : Sum  Inputs=+-  OutDataTypeStr=fixed  AccumDataTypeStr=fixed  RndMeth=Round
  Add20 : Sum  OutDataTypeStr=fixed  RndMeth=Round
  Add3 : Sum  Inputs=+-  OutDataTypeStr=fixed  AccumDataTypeStr=fixed  RndMeth=Round
  Add4 : Sum  Inputs=+-  OutDataTypeStr=fixed  AccumDataTypeStr=fixed  RndMeth=Round
  Complex to Real-Imag : ComplexToRealImag
  Complex to Real-Imag1 : ComplexToRealImag
  Constant : Constant  Commented=on  Value=1+j  OutDataTypeStr=fixdt(1,22, 15)  SampleTime=2e-8
  Constant1 : Constant  Commented=on  Value=1-j  OutDataTypeStr=fixdt(1,22, 15)  SampleTime=2e-8
  Data Type Conversion : DataTypeConversion  OutDataTypeStr=fixed  RndMeth=Round  SaturateOnIntegerOverflow=off
  Data Type Conversion1 : DataTypeConversion  OutDataTypeStr=fixed  RndMeth=Round  SaturateOnIntegerOverflow=off
  Data Type Conversion2 : DataTypeConversion  OutDataTypeStr=fixed  RndMeth=Round  SaturateOnIntegerOverflow=off
  Delay : Delay
  Delay1 : Delay
  Delay{3..14} (12 alike) : Delay  DelayLength=1
  Delay2 : Delay
  Display : Display  Commented=on
  Product : Product
  Product1 : Product
  Product2 : Product
  Real-Imag to Complex : RealImagToComplex
  Out1 : Outport
  wires:
  Delay14/1 -> Add4/2, Delay11/1
  Data Type Conversion2/1 -> Delay14/1
  Delay13/1 -> Add3/2, Add4/1
  Data Type Conversion1/1 -> Delay13/1
  Data Type Conversion/1 -> Delay12/1
  Delay12/1 -> Add3/1
  Add2/1 -> Real-Imag to Complex/2
  Delay11/1 -> Add2/2
  Delay10/1 -> Add2/1
  Delay9/1 -> Real-Imag to Complex/1
  Delay8/1 -> Product2/2
  Delay7/1 -> Product2/1
  Delay6/1 -> Product1/2
  Delay5/1 -> Product1/1
  Delay4/1 -> Product/2
  Delay3/1 -> Product/1
  Complex to Real-Imag1/2 -> Add1/2, Delay8/1
  Complex to Real-Imag/2 -> Add20/2, Delay7/1
  Complex to Real-Imag1/1 -> Add1/1, Delay6/1
  Complex to Real-Imag/1 -> Add20/1, Delay5/1
  Add1/1 -> Delay4/1
  Add20/1 -> Delay3/1
  Add3/1 -> Delay10/1
  Add4/1 -> Delay9/1
  Delay2/1 -> Data Type Conversion2/1
  Delay1/1 -> Data Type Conversion1/1
  Delay/1 -> Data Type Conversion/1
  Product2/1 -> Delay2/1
  Product1/1 -> Delay1/1
  Product/1 -> Delay/1
  x1/1 -> Complex to Real-Imag/1
  In3/1 -> Complex to Real-Imag1/1
  Real-Imag to Complex/1 -> Out1/1

== system fft_overlap_tomori/FFT64_outMuxed/64pointFFTchan/FFT64/FFT32/FFT16/complexmult2 ==
  x1 : Inport
  In3 : Inport  Port=2
  Add1 : Sum  OutDataTypeStr=addConst  RndMeth=Round
  Add2 : Sum  Inputs=+-  OutDataTypeStr=fixed  AccumDataTypeStr=fixed  RndMeth=Round
  Add20 : Sum  OutDataTypeStr=fixed  RndMeth=Round
  Add3 : Sum  Inputs=+-  OutDataTypeStr=fixed  AccumDataTypeStr=fixed  RndMeth=Round
  Add4 : Sum  Inputs=+-  OutDataTypeStr=fixed  AccumDataTypeStr=fixed  RndMeth=Round
  Complex to Real-Imag : ComplexToRealImag
  Complex to Real-Imag1 : ComplexToRealImag
  Constant : Constant  Commented=on  Value=1+j  OutDataTypeStr=fixdt(1,22, 15)  SampleTime=2e-8
  Constant1 : Constant  Commented=on  Value=1-j  OutDataTypeStr=fixdt(1,22, 15)  SampleTime=2e-8
  Data Type Conversion : DataTypeConversion  OutDataTypeStr=fixed  RndMeth=Round  SaturateOnIntegerOverflow=off
  Data Type Conversion1 : DataTypeConversion  OutDataTypeStr=fixed  RndMeth=Round  SaturateOnIntegerOverflow=off
  Data Type Conversion2 : DataTypeConversion  OutDataTypeStr=fixed  RndMeth=Round  SaturateOnIntegerOverflow=off
  Delay : Delay
  Delay1 : Delay
  Delay{3..14} (12 alike) : Delay  DelayLength=1
  Delay2 : Delay
  Display : Display  Commented=on
  Product : Product
  Product1 : Product
  Product2 : Product
  Real-Imag to Complex : RealImagToComplex
  Out1 : Outport
  wires:
  Real-Imag to Complex/1 -> Out1/1
  In3/1 -> Complex to Real-Imag1/1
  x1/1 -> Complex to Real-Imag/1
  Product/1 -> Delay/1
  Product1/1 -> Delay1/1
  Product2/1 -> Delay2/1
  Delay/1 -> Data Type Conversion/1
  Delay1/1 -> Data Type Conversion1/1
  Delay2/1 -> Data Type Conversion2/1
  Add4/1 -> Delay9/1
  Add3/1 -> Delay10/1
  Add20/1 -> Delay3/1
  Add1/1 -> Delay4/1
  Complex to Real-Imag/1 -> Delay5/1, Add20/1
  Complex to Real-Imag1/1 -> Delay6/1, Add1/1
  Complex to Real-Imag/2 -> Delay7/1, Add20/2
  Complex to Real-Imag1/2 -> Delay8/1, Add1/2
  Delay3/1 -> Product/1
  Delay4/1 -> Product/2
  Delay5/1 -> Product1/1
  Delay6/1 -> Product1/2
  Delay7/1 -> Product2/1
  Delay8/1 -> Product2/2
  Delay9/1 -> Real-Imag to Complex/1
  Delay10/1 -> Add2/1
  Delay11/1 -> Add2/2
  Add2/1 -> Real-Imag to Complex/2
  Delay12/1 -> Add3/1
  Data Type Conversion/1 -> Delay12/1
  Data Type Conversion1/1 -> Delay13/1
  Delay13/1 -> Add4/1, Add3/2
  Data Type Conversion2/1 -> Delay14/1
  Delay14/1 -> Delay11/1, Add4/2

== system fft_overlap_tomori/FFT64_outMuxed/64pointFFTchan/FFT64/FFT32/FFT16/complexmult3 ==
  x1 : Inport
  In3 : Inport  Port=2
  Add1 : Sum  OutDataTypeStr=addConst  RndMeth=Round
  Add2 : Sum  Inputs=+-  OutDataTypeStr=fixed  AccumDataTypeStr=fixed  RndMeth=Round
  Add20 : Sum  OutDataTypeStr=fixed  RndMeth=Round
  Add3 : Sum  Inputs=+-  OutDataTypeStr=fixed  AccumDataTypeStr=fixed  RndMeth=Round
  Add4 : Sum  Inputs=+-  OutDataTypeStr=fixed  AccumDataTypeStr=fixed  RndMeth=Round
  Complex to Real-Imag : ComplexToRealImag
  Complex to Real-Imag1 : ComplexToRealImag
  Constant : Constant  Commented=on  Value=1+j  OutDataTypeStr=fixdt(1,22, 15)  SampleTime=2e-8
  Constant1 : Constant  Commented=on  Value=1-j  OutDataTypeStr=fixdt(1,22, 15)  SampleTime=2e-8
  Data Type Conversion : DataTypeConversion  OutDataTypeStr=fixed  RndMeth=Round  SaturateOnIntegerOverflow=off
  Data Type Conversion1 : DataTypeConversion  OutDataTypeStr=fixed  RndMeth=Round  SaturateOnIntegerOverflow=off
  Data Type Conversion2 : DataTypeConversion  OutDataTypeStr=fixed  RndMeth=Round  SaturateOnIntegerOverflow=off
  Delay : Delay
  Delay1 : Delay
  Delay{3..14} (12 alike) : Delay  DelayLength=1
  Delay2 : Delay
  Display : Display  Commented=on
  Product : Product
  Product1 : Product
  Product2 : Product
  Real-Imag to Complex : RealImagToComplex
  Out1 : Outport
  wires:
  Delay14/1 -> Add4/2, Delay11/1
  Data Type Conversion2/1 -> Delay14/1
  Delay13/1 -> Add3/2, Add4/1
  Data Type Conversion1/1 -> Delay13/1
  Data Type Conversion/1 -> Delay12/1
  Delay12/1 -> Add3/1
  Add2/1 -> Real-Imag to Complex/2
  Delay11/1 -> Add2/2
  Delay10/1 -> Add2/1
  Delay9/1 -> Real-Imag to Complex/1
  Delay8/1 -> Product2/2
  Delay7/1 -> Product2/1
  Delay6/1 -> Product1/2
  Delay5/1 -> Product1/1
  Delay4/1 -> Product/2
  Delay3/1 -> Product/1
  Complex to Real-Imag1/2 -> Add1/2, Delay8/1
  Complex to Real-Imag/2 -> Add20/2, Delay7/1
  Complex to Real-Imag1/1 -> Add1/1, Delay6/1
  Complex to Real-Imag/1 -> Add20/1, Delay5/1
  Add1/1 -> Delay4/1
  Add20/1 -> Delay3/1
  Add3/1 -> Delay10/1
  Add4/1 -> Delay9/1
  Delay2/1 -> Data Type Conversion2/1
  Delay1/1 -> Data Type Conversion1/1
  Delay/1 -> Data Type Conversion/1
  Product2/1 -> Delay2/1
  Product1/1 -> Delay1/1
  Product/1 -> Delay/1
  x1/1 -> Complex to Real-Imag/1
  In3/1 -> Complex to Real-Imag1/1
  Real-Imag to Complex/1 -> Out1/1

== system fft_overlap_tomori/FFT64_outMuxed/64pointFFTchan/FFT64/FFT32/FFT16/multByExp(-j*Pi//4) ==
  x4 : Inport
  Add : Sum  OutDataTypeStr=fixed  RndMeth=Round
  Add1 : Sum  Inputs=+-  OutDataTypeStr=fixed  RndMeth=Round
  Complex to Real-Imag : ComplexToRealImag
  Data Type Conversion : DataTypeConversion  OutDataTypeStr=fixed  RndMeth=Round  SaturateOnIntegerOverflow=off
  Delay1 : Delay  DelayLength=1
  Delay24 : Delay  DelayLength=1
  Gain : Gain  Gain=sqrt(2)/2  ParamDataTypeStr=const
  Real-Imag to Complex : RealImagToComplex
  Out1 : Outport
  wires:
  Data Type Conversion/1 -> Delay24/1
  Delay1/1 -> Data Type Conversion/1
  Gain/1 -> Delay1/1
  Complex to Real-Imag/1 -> Add1/2, Add/1
  Complex to Real-Imag/2 -> Add1/1, Add/2
  Add/1 -> Real-Imag to Complex/1
  Add1/1 -> Real-Imag to Complex/2
  Delay24/1 -> Complex to Real-Imag/1
  Real-Imag to Complex/1 -> Out1/1
  x4/1 -> Gain/1

== system fft_overlap_tomori/FFT64_outMuxed/64pointFFTchan/FFT64/FFT32/FFT16/multByExp(-j*Pi//4)1 ==
  x4 : Inport
  Add : Sum  OutDataTypeStr=fixed  RndMeth=Round
  Add1 : Sum  Inputs=+-  OutDataTypeStr=fixed  RndMeth=Round
  Complex to Real-Imag : ComplexToRealImag
  Data Type Conversion : DataTypeConversion  OutDataTypeStr=fixed  RndMeth=Round  SaturateOnIntegerOverflow=off
  Delay1 : Delay  DelayLength=1
  Delay24 : Delay  DelayLength=1
  Gain : Gain  Gain=sqrt(2)/2  ParamDataTypeStr=const
  Real-Imag to Complex : RealImagToComplex
  Out1 : Outport
  wires:
  Data Type Conversion/1 -> Delay24/1
  Delay1/1 -> Data Type Conversion/1
  Gain/1 -> Delay1/1
  Complex to Real-Imag/1 -> Add1/2, Add/1
  Complex to Real-Imag/2 -> Add1/1, Add/2
  Add/1 -> Real-Imag to Complex/1
  Add1/1 -> Real-Imag to Complex/2
  Delay24/1 -> Complex to Real-Imag/1
  Real-Imag to Complex/1 -> Out1/1
  x4/1 -> Gain/1
